simulink model "HW2_2_disc_30"  (R2021a)
settings: Solver=VariableStepAuto  StartTime=0.0  StopTime=2  RelTol=1e-3
settings Model: Creator=jhart  LastModifiedBy=jhart

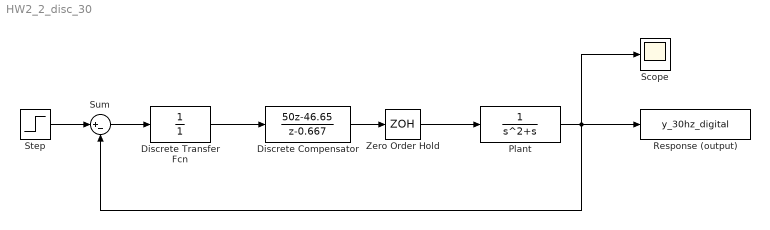
== system HW2_2_disc_30 ==
  Discrete Transfer Fcn : DiscreteTransferFcn  Denominator=[1]  SampleTime=0.033
  Discrete Compensator : DiscreteTransferFcn  Numerator=[50 -46.65]  Denominator=[1 -0.667]  SampleTime=0.033
  Plant : TransferFcn  Denominator=[1 1 0]
  Response (output) : ToWorkspace  VariableName=y_30hz_digital  SaveFormat=Timeseries  SampleTime=0.033
  Scope : Scope
  Step : Step  Time=0  SampleTime=0
  Sum : Sum  Inputs=|+-
  Zero Order Hold : ZeroOrderHold  SampleTime=0.033
  wires:
  Plant/1 -> Scope/1, Sum/2, Response (output)/1
  Step/1 -> Sum/1
  Discrete Transfer Fcn/1 -> Discrete Compensator/1
  Discrete Compensator/1 -> Zero Order Hold/1
  Zero Order Hold/1 -> Plant/1
  Sum/1 -> Discrete Transfer Fcn/1
